simulink model "Alberta_Grid_138kV_240kV_500kV"  (R2024b)
(part 2 of 2)

  PV36 : PMComponent  Tag=PSATblock  Description=Power Flow  PhysicalDomain=psatdomain  LeftPortType=p1  RightPortType=p1  RConnTagsString=__newr0  mask(PV){p2_3q=[1000  100], p4q=0.32, p5q=1.00, p6_7q=[0.8  -0.2], p8_9q=[1.1  0.9], p10q=1, p11q=on}
      mask prompts: p2_3q "Power and Voltage Ratings [MVA, kV]"; p4q "Active Power [p.u.]"; p5q "Voltage Magnitude [p.u.]"; p6_7q "Qmax and Qmin [p.u.  p.u.]"; p8_9q "Vmax and Vmin [p.u.  p.u.]"; p10q "Loss Participation Factor"; p11q "Connected"
      mask help:
      | This block defines a PV bus for load flow studies:
      |
      | P = Pcost.
      | V = Vdes.
      mask init:
      | [x,y] = fm_draw('circle');
      | [xp,yp] = fm_draw('P');
      mask Callback p11q: fm_block
      mask Display:
      | plot(x,y)
      | color('blue')
      | plot(0.3*xp-0.35,0.6*yp,[0.1 0.3 0.5],[0.3 -0.3 0.3])
  PV37 : PMComponent  Tag=PSATblock  Description=Power Flow  PhysicalDomain=psatdomain  LeftPortType=p1  RightPortType=p1  RConnTagsString=__newr0  mask(PV){p2_3q=[1000  100], p4q=0.03, p5q=1.00, p6_7q=[0.8  -0.2], p8_9q=[1.1  0.9], p10q=1, p11q=on}
      mask prompts: p2_3q "Power and Voltage Ratings [MVA, kV]"; p4q "Active Power [p.u.]"; p5q "Voltage Magnitude [p.u.]"; p6_7q "Qmax and Qmin [p.u.  p.u.]"; p8_9q "Vmax and Vmin [p.u.  p.u.]"; p10q "Loss Participation Factor"; p11q "Connected"
      mask help:
      | This block defines a PV bus for load flow studies:
      |
      | P = Pcost.
      | V = Vdes.
      mask init:
      | [x,y] = fm_draw('circle');
      | [xp,yp] = fm_draw('P');
      mask Callback p11q: fm_block
      mask Display:
      | plot(x,y)
      | color('blue')
      | plot(0.3*xp-0.35,0.6*yp,[0.1 0.3 0.5],[0.3 -0.3 0.3])
  PV38 : PMComponent  Tag=PSATblock  Description=Power Flow  PhysicalDomain=psatdomain  LeftPortType=p1  RightPortType=p1  RConnTagsString=__newr0  mask(PV){p2_3q=[1000  100], p4q=0.049, p5q=1.00, p6_7q=[0.8  -0.2], p8_9q=[1.1  0.9], p10q=1, p11q=on}
      mask prompts: p2_3q "Power and Voltage Ratings [MVA, kV]"; p4q "Active Power [p.u.]"; p5q "Voltage Magnitude [p.u.]"; p6_7q "Qmax and Qmin [p.u.  p.u.]"; p8_9q "Vmax and Vmin [p.u.  p.u.]"; p10q "Loss Participation Factor"; p11q "Connected"
      mask help:
      | This block defines a PV bus for load flow studies:
      |
      | P = Pcost.
      | V = Vdes.
      mask init:
      | [x,y] = fm_draw('circle');
      | [xp,yp] = fm_draw('P');
      mask Callback p11q: fm_block
      mask Display:
      | plot(x,y)
      | color('blue')
      | plot(0.3*xp-0.35,0.6*yp,[0.1 0.3 0.5],[0.3 -0.3 0.3])
  PV39 : PMComponent  Tag=PSATblock  Description=Power Flow  PhysicalDomain=psatdomain  LeftPortType=p1  RightPortType=p1  RConnTagsString=__newr0  mask(PV){p2_3q=[1000  100], p4q=0.059054, p5q=1.00, p6_7q=[0.8  -0.2], p8_9q=[1.1  0.9], p10q=1, p11q=on}
      mask prompts: p2_3q "Power and Voltage Ratings [MVA, kV]"; p4q "Active Power [p.u.]"; p5q "Voltage Magnitude [p.u.]"; p6_7q "Qmax and Qmin [p.u.  p.u.]"; p8_9q "Vmax and Vmin [p.u.  p.u.]"; p10q "Loss Participation Factor"; p11q "Connected"
      mask help:
      | This block defines a PV bus for load flow studies:
      |
      | P = Pcost.
      | V = Vdes.
      mask init:
      | [x,y] = fm_draw('circle');
      | [xp,yp] = fm_draw('P');
      mask Callback p11q: fm_block
      mask Display:
      | plot(x,y)
      | color('blue')
      | plot(0.3*xp-0.35,0.6*yp,[0.1 0.3 0.5],[0.3 -0.3 0.3])
  PV4 : PMComponent  Tag=PSATblock  Description=Power Flow  PhysicalDomain=psatdomain  LeftPortType=p1  RightPortType=p1  RConnTagsString=__newr0  mask(PV){p2_3q=[1000  100], p4q=0.149, p5q=1.00, p6_7q=[0.8  -0.2], p8_9q=[1.1  0.9], p10q=1, p11q=on}
      mask prompts: p2_3q "Power and Voltage Ratings [MVA, kV]"; p4q "Active Power [p.u.]"; p5q "Voltage Magnitude [p.u.]"; p6_7q "Qmax and Qmin [p.u.  p.u.]"; p8_9q "Vmax and Vmin [p.u.  p.u.]"; p10q "Loss Participation Factor"; p11q "Connected"
      mask help:
      | This block defines a PV bus for load flow studies:
      |
      | P = Pcost.
      | V = Vdes.
      mask init:
      | [x,y] = fm_draw('circle');
      | [xp,yp] = fm_draw('P');
      mask Callback p11q: fm_block
      mask Display:
      | plot(x,y)
      | color('blue')
      | plot(0.3*xp-0.35,0.6*yp,[0.1 0.3 0.5],[0.3 -0.3 0.3])
  PV40 : PMComponent  Tag=PSATblock  Description=Power Flow  PhysicalDomain=psatdomain  LeftPortType=p1  RightPortType=p1  RConnTagsString=__newr0  mask(PV){p2_3q=[1000  100], p4q=1.038, p5q=1.00, p6_7q=[0.8  -0.2], p8_9q=[1.1  0.9], p10q=1, p11q=on}
      mask prompts: p2_3q "Power and Voltage Ratings [MVA, kV]"; p4q "Active Power [p.u.]"; p5q "Voltage Magnitude [p.u.]"; p6_7q "Qmax and Qmin [p.u.  p.u.]"; p8_9q "Vmax and Vmin [p.u.  p.u.]"; p10q "Loss Participation Factor"; p11q "Connected"
      mask help:
      | This block defines a PV bus for load flow studies:
      |
      | P = Pcost.
      | V = Vdes.
      mask init:
      | [x,y] = fm_draw('circle');
      | [xp,yp] = fm_draw('P');
      mask Callback p11q: fm_block
      mask Display:
      | plot(x,y)
      | color('blue')
      | plot(0.3*xp-0.35,0.6*yp,[0.1 0.3 0.5],[0.3 -0.3 0.3])
  PV41 : PMComponent  Tag=PSATblock  Description=Power Flow  PhysicalDomain=psatdomain  LeftPortType=p1  RightPortType=p1  RConnTagsString=__newr0  mask(PV){p2_3q=[1000  100], p4q=0.0864375, p5q=1.00, p6_7q=[0.8  -0.2], p8_9q=[1.1  0.9], p10q=1, p11q=on}
      mask prompts: p2_3q "Power and Voltage Ratings [MVA, kV]"; p4q "Active Power [p.u.]"; p5q "Voltage Magnitude [p.u.]"; p6_7q "Qmax and Qmin [p.u.  p.u.]"; p8_9q "Vmax and Vmin [p.u.  p.u.]"; p10q "Loss Participation Factor"; p11q "Connected"
      mask help:
      | This block defines a PV bus for load flow studies:
      |
      | P = Pcost.
      | V = Vdes.
      mask init:
      | [x,y] = fm_draw('circle');
      | [xp,yp] = fm_draw('P');
      mask Callback p11q: fm_block
      mask Display:
      | plot(x,y)
      | color('blue')
      | plot(0.3*xp-0.35,0.6*yp,[0.1 0.3 0.5],[0.3 -0.3 0.3])
  PV5 : PMComponent  Tag=PSATblock  Description=Power Flow  PhysicalDomain=psatdomain  LeftPortType=p1  RightPortType=p1  RConnTagsString=__newr0  mask(PV){p2_3q=[1000  100], p4q=0.072, p5q=1.00, p6_7q=[0.8  -0.2], p8_9q=[1.1  0.9], p10q=1, p11q=on}
      mask prompts: p2_3q "Power and Voltage Ratings [MVA, kV]"; p4q "Active Power [p.u.]"; p5q "Voltage Magnitude [p.u.]"; p6_7q "Qmax and Qmin [p.u.  p.u.]"; p8_9q "Vmax and Vmin [p.u.  p.u.]"; p10q "Loss Participation Factor"; p11q "Connected"
      mask help:
      | This block defines a PV bus for load flow studies:
      |
      | P = Pcost.
      | V = Vdes.
      mask init:
      | [x,y] = fm_draw('circle');
      | [xp,yp] = fm_draw('P');
      mask Callback p11q: fm_block
      mask Display:
      | plot(x,y)
      | color('blue')
      | plot(0.3*xp-0.35,0.6*yp,[0.1 0.3 0.5],[0.3 -0.3 0.3])
  PV6 : PMComponent  Tag=PSATblock  Description=Power Flow  PhysicalDomain=psatdomain  LeftPortType=p1  RightPortType=p1  RConnTagsString=__newr0  mask(PV){p2_3q=[1000  100], p4q=0.3, p5q=1.00, p6_7q=[0.8  -0.2], p8_9q=[1.1  0.9], p10q=1, p11q=on}
      mask prompts: p2_3q "Power and Voltage Ratings [MVA, kV]"; p4q "Active Power [p.u.]"; p5q "Voltage Magnitude [p.u.]"; p6_7q "Qmax and Qmin [p.u.  p.u.]"; p8_9q "Vmax and Vmin [p.u.  p.u.]"; p10q "Loss Participation Factor"; p11q "Connected"
      mask help:
      | This block defines a PV bus for load flow studies:
      |
      | P = Pcost.
      | V = Vdes.
      mask init:
      | [x,y] = fm_draw('circle');
      | [xp,yp] = fm_draw('P');
      mask Callback p11q: fm_block
      mask Display:
      | plot(x,y)
      | color('blue')
      | plot(0.3*xp-0.35,0.6*yp,[0.1 0.3 0.5],[0.3 -0.3 0.3])
  PV7 : PMComponent  Tag=PSATblock  Description=Power Flow  PhysicalDomain=psatdomain  LeftPortType=p1  RightPortType=p1  RConnTagsString=__newr0  mask(PV){p2_3q=[1000  100], p4q=0.421, p5q=1.00, p6_7q=[0.8  -0.2], p8_9q=[1.1  0.9], p10q=1, p11q=on}
      mask prompts: p2_3q "Power and Voltage Ratings [MVA, kV]"; p4q "Active Power [p.u.]"; p5q "Voltage Magnitude [p.u.]"; p6_7q "Qmax and Qmin [p.u.  p.u.]"; p8_9q "Vmax and Vmin [p.u.  p.u.]"; p10q "Loss Participation Factor"; p11q "Connected"
      mask help:
      | This block defines a PV bus for load flow studies:
      |
      | P = Pcost.
      | V = Vdes.
      mask init:
      | [x,y] = fm_draw('circle');
      | [xp,yp] = fm_draw('P');
      mask Callback p11q: fm_block
      mask Display:
      | plot(x,y)
      | color('blue')
      | plot(0.3*xp-0.35,0.6*yp,[0.1 0.3 0.5],[0.3 -0.3 0.3])
  PV8 : PMComponent  Tag=PSATblock  Description=Power Flow  PhysicalDomain=psatdomain  LeftPortType=p1  RightPortType=p1  RConnTagsString=__newr0  mask(PV){p2_3q=[1000  100], p4q=0.1, p5q=1.00, p6_7q=[0.8  -0.2], p8_9q=[1.1  0.9], p10q=1, p11q=on}
      mask prompts: p2_3q "Power and Voltage Ratings [MVA, kV]"; p4q "Active Power [p.u.]"; p5q "Voltage Magnitude [p.u.]"; p6_7q "Qmax and Qmin [p.u.  p.u.]"; p8_9q "Vmax and Vmin [p.u.  p.u.]"; p10q "Loss Participation Factor"; p11q "Connected"
      mask help:
      | This block defines a PV bus for load flow studies:
      |
      | P = Pcost.
      | V = Vdes.
      mask init:
      | [x,y] = fm_draw('circle');
      | [xp,yp] = fm_draw('P');
      mask Callback p11q: fm_block
      mask Display:
      | plot(x,y)
      | color('blue')
      | plot(0.3*xp-0.35,0.6*yp,[0.1 0.3 0.5],[0.3 -0.3 0.3])
  PV9 : PMComponent  Tag=PSATblock  Description=Power Flow  PhysicalDomain=psatdomain  LeftPortType=p1  RightPortType=p1  RConnTagsString=__newr0  mask(PV){p2_3q=[1000  100], p4q=0.009, p5q=1.00, p6_7q=[0.8  -0.2], p8_9q=[1.1  0.9], p10q=1, p11q=on}
      mask prompts: p2_3q "Power and Voltage Ratings [MVA, kV]"; p4q "Active Power [p.u.]"; p5q "Voltage Magnitude [p.u.]"; p6_7q "Qmax and Qmin [p.u.  p.u.]"; p8_9q "Vmax and Vmin [p.u.  p.u.]"; p10q "Loss Participation Factor"; p11q "Connected"
      mask help:
      | This block defines a PV bus for load flow studies:
      |
      | P = Pcost.
      | V = Vdes.
      mask init:
      | [x,y] = fm_draw('circle');
      | [xp,yp] = fm_draw('P');
      mask Callback p11q: fm_block
      mask Display:
      | plot(x,y)
      | color('blue')
      | plot(0.3*xp-0.35,0.6*yp,[0.1 0.3 0.5],[0.3 -0.3 0.3])
  Slack : PMComponent  Tag=PSATblock  Description=Power Flow  PhysicalDomain=psatdomain  LeftPortType=p1  RightPortType=p1  RConnTagsString=__newr0  mask(SW){p2_3q=[1000  100], p4q=1.00, p5q=0.00, p6_7q=[1.5  -1.5], p8_9q=[1.1  0.9], p10q=1.54853, p11q=1, p12q=on, p13q=on}
      mask prompts: p2_3q "Power and Voltage Ratings [MVA, kV]"; p4q "Voltage Magnitude [p.u.]"; p5q "Reference Phase Angle [rad]"; p6_7q "Qmax and Qmin [p.u.  p.u.]"; p8_9q "Vmax and Vmin  [p.u.  p.u.]"; p10q "Active Power Guess [p.u.]"; p11q "Loss Participation Factor"; p12q "Reference bus"; p13q "Connected"
      mask help:
      | This block defines a V-theta bus:
      |
      | V = V_des
      | theta = theta_des
      mask init:
      | [x,y] = fm_draw('circle');
      | [xt,yt] = fm_draw('theta');
      mask Callback p12q: fm_block
      mask Callback p13q: fm_block
      mask Display: plot([0 1 1 0 0],[0 0 1 1 0]), color('blue'), plot([0 1],[0 1],[0 1],[1 0],[0.5 1 0.5 0 0.5],[0 0.5 1 0.5 0])
  connections:
  PV2/RConn1 -- Bus17/LConn1
  PQ1/LConn1 -- Bus17/RConn1
  Line1/LConn1 -- Bus17/RConn3
  Line/RConn1 -- Bus18/RConn2
  Line/LConn1 -- Bus17/RConn2
  PQ2/LConn1 -- Bus18/RConn1
  PQ3/LConn1 -- Bus25/RConn1
  PV3/RConn1 -- Bus25/LConn1
  Line1/RConn1 -- Bus19/RConn1
  Line4/RConn1 -- Bus19/RConn2
  Line4/LConn1 -- Bus25/RConn3
  PV5/RConn1 -- Bus19/LConn1
  PQ4/LConn1 -- Bus19/RConn6
  PV4/RConn1 -- Bus 27/LConn1
  PQ5/LConn1 -- Bus 27/RConn1
  PQ35/LConn1 -- Bus 28/RConn1
  Bus 28/LConn1 -- PV14/RConn1
  PQ7/LConn1 -- Bus 22/RConn1
  Bus 22/LConn1 -- PV6/RConn1
  PQ13/LConn1 -- Bus 24/RConn1
  PQ8/LConn1 -- Bus 20/RConn1
  PV7/RConn1 -- Bus 20/LConn1
  PQ9/LConn1 -- Bus 23/RConn1
  Bus 23/LConn1 -- PV8/RConn1
  PQ10/LConn1 -- Bus 21/RConn1
  PV9/RConn1 -- Bus 21/LConn1
  Bus 27/RConn2 -- Line5/RConn1
  Line6/LConn1 -- Bus 27/RConn4
  Bus 27/RConn3 -- Line7/LConn1
  PQ34/LConn1 -- Bus 33/RConn1
  PV12/RConn1 -- Bus 33/LConn1
  Bus25/RConn4 -- Line5/LConn1
  Bus 28/RConn2 -- Line6/RConn1
  Line7/RConn1 -- Bus 33/RConn2
  Bus 28/RConn3 -- Line8/RConn1
  Line9/LConn1 -- Bus19/RConn5
  Bus 23/RConn2 -- Line10/RConn1
  Bus 21/RConn2 -- Line11/RConn1
  Bus 20/RConn2 -- Line9/RConn1
  Line10/LConn1 -- Bus19/RConn4
  Line11/LConn1 -- Bus19/RConn3
  Line13/LConn1 -- Bus 20/RConn3
  Line12/LConn1 -- Bus 20/RConn4
  Bus 22/RConn2 -- Line13/RConn1
  Bus 21/RConn3 -- Line14/RConn1
  Line14/LConn1 -- Bus 23/RConn4
  Line12/RConn1 -- Bus 23/RConn3
  Line15/LConn1 -- Bus 23/RConn5
  Bus 22/RConn3 -- Line15/RConn1
  Line16/LConn1 -- Bus 23/RConn6
  Bus 26/RConn2 -- Line16/RConn1
  Line17/LConn1 -- Bus 23/RConn7
  Bus 24/RConn2 -- Line17/RConn1
  Line8/LConn1 -- Bus25/RConn5
  Line19/LConn1 -- Bus25/RConn2
  Bus 21/RConn5 -- Line18/LConn1
  Line19/RConn1 -- Bus 21/RConn4
  PQ11/LConn1 -- Bus 26/RConn1
  PV10/RConn1 -- Bus 26/LConn1
  Line18/RConn1 -- Bus 26/RConn3
  Line20/LConn1 -- Bus 26/RConn4
  Bus 24/RConn3 -- Line20/RConn1
  Bus 22/RConn4 -- Line23/RConn1
  Bus 29/RConn2 -- Line22/RConn1
  Line22/LConn1 -- Bus 24/RConn4
  Line23/LConn1 -- Bus 24/RConn5
  PQ14/LConn1 -- Bus 29/RConn1
  Bus 29/LConn1 -- PV13/RConn1
  Bus 40/RConn2 -- Line25/RConn1
  Line26/LConn1 -- Bus 29/RConn3
  Line25/LConn1 -- Bus 29/RConn4
  Bus 30/RConn2 -- Line26/RConn1
  PQ33/LConn1 -- Bus 56/RConn1
  PQ32/LConn1 -- Bus 13/RConn1
  PV16/RConn1 -- Bus 13/LConn1
  PQ31/LConn1 -- Bus 32/RConn1
  PV17/RConn1 -- Bus 32/LConn1
  PQ30/LConn1 -- Bus 37/RConn1
  PV38/RConn1 -- Bus 37/LConn1
  PQ29/LConn1 -- Bus 36/RConn1
  PV34/RConn1 -- Bus 36/LConn1
  PQ22/LConn1 -- Bus 42/RConn1
  PV33/RConn1 -- Bus 42/LConn1
  PQ21/LConn1 -- Bus 60/RConn1
  PV32/RConn1 -- Bus 60/LConn1
  PQ20/LConn1 -- Bus 31/RConn1
  PV31/RConn1 -- Bus 31/LConn1
  Line28/LConn1 -- Bus 28/RConn4
  Bus 56/RConn2 -- Line28/RConn1
  Line29/LConn1 -- Bus 28/RConn5
  Bus 13/RConn2 -- Line29/RConn1
  Line33/LConn1 -- Bus 56/RConn3
  Bus 13/RConn3 -- Line33/RConn1
  Line35/LConn1 -- Bus 56/RConn4
  Bus 36/RConn2 -- Line35/RConn1
  Bus 31/RConn2 -- Line36/RConn1
  Line36/LConn1 -- Bus 56/RConn5
  Bus 13/RConn4 -- Line37/LConn1
  Line37/RConn1 -- Bus 32/RConn2
  Bus 32/RConn3 -- Line38/LConn1
  Line38/RConn1 -- Bus 37/RConn2
  Line39/LConn1 -- Bus 32/RConn4
  Line39/RConn1 -- Bus 36/RConn3
  Line40/LConn1 -- Bus 37/RConn3
  Bus 36/RConn4 -- Line40/RConn1
  Bus 42/RConn2 -- Line41/RConn1
  Line41/LConn1 -- Bus 37/RConn4
  Line43/RConn1 -- Bus 42/RConn3
  Line43/LConn1 -- Bus 36/RConn5
  PQ23/LConn1 -- Bus 40/RConn1
  PQ24/LConn1 -- Bus 30/RConn1
  PQ25/LConn1 -- Bus 34/RConn1
  Bus 34/LConn1 -- PV24/RConn1
  PV23/RConn1 -- Bus 30/LConn1
  Bus 40/LConn1 -- PV22/RConn1
  Line45/RConn1 -- Bus 40/RConn3
  Line45/LConn1 -- Bus 26/RConn5
  Line46/LConn1 -- Bus 27/RConn5
  Line46/RConn1 -- Bus 40/RConn4
  Bus 30/RConn3 -- Line47/RConn1
  Bus 40/RConn6 -- Line47/LConn1
  Bus 40/RConn5 -- Line49/LConn1
  Line49/RConn1 -- Bus 60/RConn3
  Line51/RConn1 -- Bus 35/RConn2
  Line51/LConn1 -- Bus 30/RConn4
  Line54/LConn1 -- Bus 34/RConn2
  Bus 38/RConn3 -- Line54/RConn1
  Bus 38/RConn1 -- PQ26/LConn1
  PQ27/LConn1 -- Bus 39/RConn1
  PV26/RConn1 -- Bus 39/LConn1
  PV27/RConn1 -- Bus 35/LConn1
  PQ28/LConn1 -- Bus 35/RConn4
  Line56/RConn1 -- Bus 39/RConn2
  Line55/RConn1 -- Bus 35/RConn3
  Bus 38/RConn4 -- Line55/LConn1
  Line56/LConn1 -- Bus 38/RConn2
  Line57/RConn1 -- Bus 35/RConn5
  Bus 39/RConn3 -- Line57/LConn1
  Bus 35/RConn6 -- Line60/RConn1
  Line59/LConn1 -- Bus 42/RConn4
  Line59/RConn1 -- Bus 35/RConn1
  Line60/LConn1 -- Bus 31/RConn3
  Line61/RConn1 -- Bus 31/RConn4
  Bus 60/RConn4 -- Line61/LConn1
  Line62/LConn1 -- Bus 33/RConn3
  Line62/RConn1 -- Bus 60/RConn2
  PV30/RConn1 -- Bus 43/LConn1
  PQ19/LConn1 -- Bus 43/RConn1
  PV29/RConn1 -- Bus 45/LConn1
  PQ18/LConn1 -- Bus 45/RConn1
  PV28/RConn1 -- Bus 47/LConn1
  PQ17/LConn1 -- Bus 47/RConn1
  PV21/RConn1 -- Bus 48/LConn1
  PQ16/LConn1 -- Bus 48/RConn1
  PV20/RConn1 -- Bus 49/LConn1
  PQ15/LConn1 -- Bus 49/RConn1
  PV19/RConn1 -- Bus 52/LConn1
  PQ12/LConn1 -- Bus 52/RConn1
  PV18/RConn1 -- Bus 4/LConn1
  PQ6/LConn1 -- Bus 4/RConn1
  PV35/RConn1 -- Bus 54/LConn1
  Bus 54/RConn1 -- PQ36/LConn1
  PV36/RConn1 -- Bus 44/LConn1
  PQ37/LConn1 -- Bus 44/RConn1
  PV37/RConn1 -- Bus 57/LConn1
  PQ38/LConn1 -- Bus 57/RConn1
  Slack/RConn1 -- Bus 6/LConn1
  PQ39/LConn1 -- Bus 6/RConn1
  PQ40/LConn1 -- Bus 46/RConn1
  PV39/RConn1 -- Bus 46/LConn1
  PQ41/LConn1 -- Bus 53/RConn1
  PV40/RConn1 -- Bus 53/LConn1
  PQ42/LConn1 -- Bus 55/RConn1
  PV41/RConn1 -- Bus 55/LConn1
  Line63/LConn1 -- Bus 42/RConn5
  Bus 43/RConn2 -- Line63/RConn1
  Line65/LConn1 -- Bus 43/RConn3
  Line65/RConn1 -- Bus 47/RConn2
  Line68/RConn1 -- Bus 48/RConn2
  Line68/LConn1 -- Bus 42/RConn6
  Bus 45/RConn5 -- Line70/LConn1
  Line70/RConn1 -- Bus 47/RConn3
  Line71/RConn1 -- Bus 49/RConn2
  Bus 45/RConn4 -- Line71/LConn1
  Line73/LConn1 -- Bus 45/RConn3
  Bus 6/RConn2 -- Line72/RConn1
  Line72/LConn1 -- Bus 45/RConn2
  Bus 46/RConn2 -- Line73/RConn1
  Line74/RConn1 -- Bus 48/RConn4
  Bus 47/RConn4 -- Line74/LConn1
  Bus 47/RConn5 -- Line75/LConn1
  Line75/RConn1 -- Bus 49/RConn3
  Line76/RConn1 -- Bus 52/RConn2
  Bus 47/RConn6 -- Line76/LConn1
  Line77/RConn1 -- Bus 4/RConn2
  Line77/LConn1 -- Bus 48/RConn3
  Bus 49/RConn5 -- Line79/LConn1
  Line79/RConn1 -- Bus 54/RConn2
  Line80/LConn1 -- Bus 49/RConn4
  Bus 53/RConn2 -- Line80/RConn1
  Line81/LConn1 -- Bus 49/RConn6
  Bus 46/RConn3 -- Line81/RConn1
  Bus 52/RConn4 -- Line82/LConn1
  Line82/RConn1 -- Bus 4/RConn3
  Line83/RConn1 -- Bus 54/RConn3
  Line83/LConn1 -- Bus 52/RConn3
  Bus 53/RConn3 -- Line86/RConn1
  Line87/RConn1 -- Bus 55/RConn2
  Line86/LConn1 -- Bus 54/RConn4
  Line87/LConn1 -- Bus 54/RConn5
  Line88/LConn1 -- Bus 39/RConn4
  Bus 44/RConn2 -- Line88/RConn1
  Line92/LConn1 -- Bus 44/RConn3
  Bus 6/RConn3 -- Line92/RConn1
  Bus 6/RConn4 -- Line94/LConn1
  Line94/RConn1 -- Bus 46/RConn4
  Line95/LConn1 -- Bus 57/RConn2
  Line95/RConn1 -- Bus 6/RConn5
  Bus 53/RConn4 -- Line96/RConn1
  Line96/LConn1 -- Bus 46/RConn5
  Bus 53/RConn5 -- Line97/LConn1
  Line97/RConn1 -- Bus 55/RConn3
  Line2/RConn1 -- Bus 4/RConn4
  Line2/LConn1 -- Bus 47/RConn7
  Bus 44/RConn4 -- Line3/LConn1
  Line3/RConn1 -- Bus 53/RConn6
  PV1/RConn1 -- Bus 38/LConn1
